simulink model "nepr"  (R2018b)
settings: Solver=FixedStepAuto  StartTime=0.0  StopTime=10.0  FixedStep=0.00001  RelTol=1e-3
settings Model: Creator=Еня  LastModifiedBy=Еня

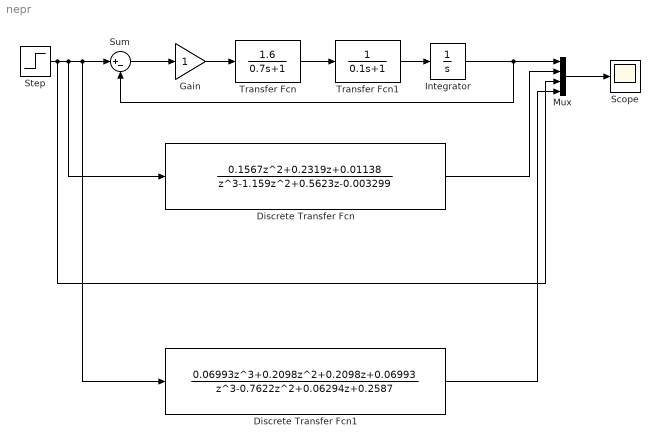
== system nepr ==
  Discrete Transfer Fcn : DiscreteTransferFcn  Numerator=[0.1567 0.2319 0.01138]  Denominator=[1 -1.159 0.5623 -0.003299]  SampleTime=0.5
  Discrete Transfer Fcn1 : DiscreteTransferFcn  Numerator=[0.06993 0.2098 0.2098 0.06993]  Denominator=[1 -0.7622 0.06294 0.2587]  SampleTime=0.5
  Gain : Gain
  Integrator : Integrator
  Mux : Mux
  Scope : Scope
  Step : Step  Time=0  SampleTime=0
  Sum : Sum  Inputs=|+-
  Transfer Fcn : TransferFcn  Numerator=[1.6]  Denominator=[0.7 1]
  Transfer Fcn1 : TransferFcn  Denominator=[0.1 1]
  wires:
  Step/1 -> Mux/3, Discrete Transfer Fcn1/1, Sum/1, Discrete Transfer Fcn/1
  Sum/1 -> Gain/1
  Gain/1 -> Transfer Fcn/1
  Transfer Fcn/1 -> Transfer Fcn1/1
  Transfer Fcn1/1 -> Integrator/1
  Integrator/1 -> Mux/1, Sum/2
  Mux/1 -> Scope/1
  Discrete Transfer Fcn/1 -> Mux/2
  Discrete Transfer Fcn1/1 -> Mux/4
